simulink model "BPSK_FS_CFO_STO_finial"  (R2014b)
settings: Solver=VariableStepDiscrete  StartTime=0.0  StopTime=inf  RelTol=1e-3
values from neighbouring files (symbols this model uses):
  L = length(corr)    [barkerBits.m]
undefined symbols (not defined in the file or in its folder): alpha, del_f, dfilt, jsin, N, timing_offset, Ts
libraries: commnoisgen2 x4, commdigbbndpm3 x2, dspindex x2, dspobslib x2, dspsigops x2, commfilt2 x2, commchan3 x1, commrandsrc2 x1, simulink x1, commsink2 x1
settings Model: Creator=magarini_2  LastModifiedBy=magarini_2
settings OptimizationCC: UseDivisionForNetSlopeComputation=off  SimCompilerOptimization=off
settings DebuggingCC: FrameProcessingCompatibilityMsg=error
settings RTWCC: RTWCompilerOptimization=off

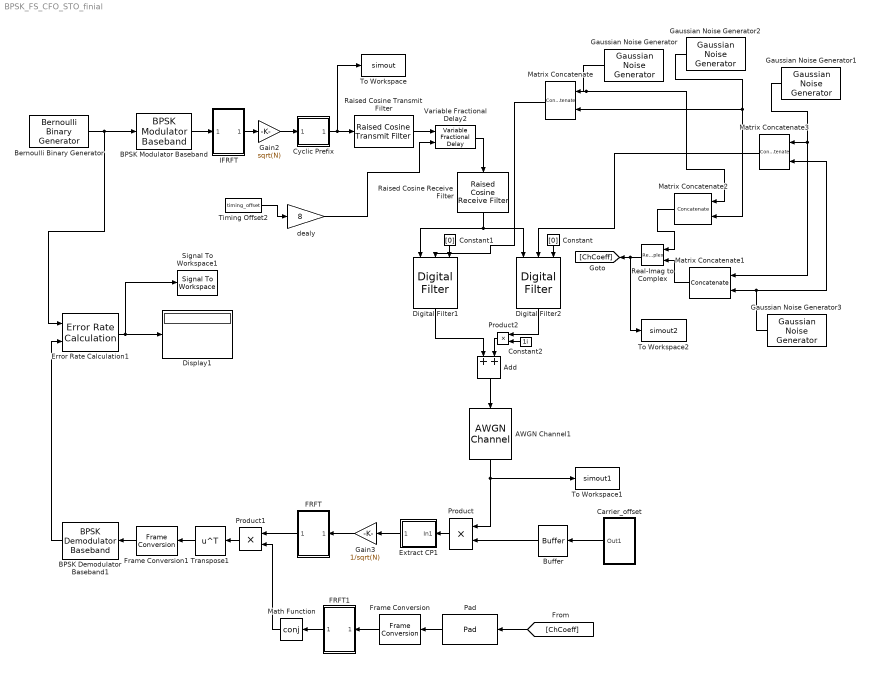
== system BPSK_FS_CFO_STO_finial ==
  AWGN Channel1 : commchan3/AWGN Channel  InputProcessing=Columns as channels (frame based)  seed=67  noiseMode="Signal to noise ratio  (SNR)"  EbNodB=50  EsNodB=10  SNRdB=SNR  bitsPerSym=1  Ps=1  Tsym=1  variance=1
  Add : Sum
  BPSK Demodulator Baseband1 : commdigbbndpm3/BPSK Demodulator Baseband  Ph=0  DecType=Hard decision  VarSource=Dialog  Variance=1  outDtype=Inherit via internal rule  derotateFactorWordLen=16
  BPSK Modulator Baseband : commdigbbndpm3/BPSK Modulator Baseband  Ph=0  outDtype=double  outWordLen=16  outUDDataType=sfix(16)  outFracLenMode=Best precision  outFracLen=15
  Bernoulli Binary Generator : commrandsrc2/Bernoulli Binary Generator  P=.5  seed=1361  Ts=Ts/N  frameBased=on  sampPerFrame=N  orient=off  outDataType=double
  Buffer : Buffer  N=N+L  TreatMby1Signals=One channel
  Carrier_offset : Subsystem
  Constant : Constant  Value=[0]  VectorParams1D=off  FramePeriod=1
      settings: SamplingMode=Frame based
  Constant1 : Constant  Value=[0]  VectorParams1D=off  FramePeriod=1
      settings: SamplingMode=Frame based
  Constant2 : Constant  Value=1i
  Cyclic Prefix : Subsystem
      mask Display: disp('CP')
  Digital Filter1 : dspobslib/Digital Filter  TypePopup=IIR (poles & zeros)  IIRFiltStruct=Direct form II transposed  AllPoleFiltStruct=Direct form  FIRFiltStruct=Direct form  CoeffSource=Input port(s)  NumCoeffs=randn  DenCoeffs=[1 1]  BiQuadCoeffs=[1 0.3 0.4 1 0.1 0.2]  LatticeCoeffs=[0.2 0.4]  denIgnore=on  FiltPerSampPopup=One filter per frame  IC=0  ICnum=0  ICden=0  roundingMode=Floor  overflowMode=off  ScaleValues=1  scaleValueFracLength=14  stageInFracLength=15  stageOutFracLength=15  FilterSource=Input port(s)  dfiltObjectName=dfilt.dffir([1 2 1])  InputProcessing=Columns as channels (frame based)
  Digital Filter2 : dspobslib/Digital Filter  TypePopup=IIR (poles & zeros)  IIRFiltStruct=Direct form II transposed  AllPoleFiltStruct=Direct form  FIRFiltStruct=Direct form  CoeffSource=Input port(s)  NumCoeffs=randn  DenCoeffs=[1 1]  BiQuadCoeffs=[1 0.3 0.4 1 0.1 0.2]  LatticeCoeffs=[0.2 0.4]  denIgnore=on  FiltPerSampPopup=One filter per frame  IC=0  ICnum=0  ICden=0  roundingMode=Floor  overflowMode=off  ScaleValues=1  scaleValueFracLength=14  stageInFracLength=15  stageOutFracLength=15  FilterSource=Input port(s)  dfiltObjectName=dfilt.dffir([1 2 1])  InputProcessing=Columns as channels (frame based)
  Display1 : Display
  Error Rate Calculation1 : commsink2/Error Rate Calculation  N=N  st_delay=N  cp_mode=Entire frame  subframe=[]  PMode=Port  WsName=ErrorVec  RsMode2=off  stop=on  numErr=maxNumErrs  maxBits=maxNumBits
  Extract CP1 : Subsystem
      mask Display: disp('CP^{-1}')
  FRFT : Subsystem
  FRFT1 : Subsystem
  Frame Conversion : FrameConversion  OutFrame=Sample-based
  Frame Conversion1 : FrameConversion
  Gain2 : Gain  Gain=sqrt(N)  OutDataTypeStr=double
  Gain3 : Gain  Gain=1/sqrt(N)
  Gaussian Noise Generator : commnoisgen2/Gaussian Noise Generator  m=0  d=1/4  s=1772  Ts=1  frameBased=on  sampPerFrame=1  orient=off  outDataType=double
  Gaussian Noise Generator1 : commnoisgen2/Gaussian Noise Generator  m=0  d=1/4  s=12313  Ts=1  frameBased=on  sampPerFrame=1  orient=off  outDataType=double
  Gaussian Noise Generator2 : commnoisgen2/Gaussian Noise Generator  m=0  d=1/4  s=14123  Ts=1  frameBased=on  sampPerFrame=1  orient=off  outDataType=double
  Gaussian Noise Generator3 : commnoisgen2/Gaussian Noise Generator  m=0  d=1/4  s=6632  Ts=1  frameBased=on  sampPerFrame=1  orient=off  outDataType=double
  IFRFT : Subsystem
  Math Function : Math  Operator=conj  SaturateOnIntegerOverflow=on
  Matrix Concatenate : Concatenate  Mode=Multidimensional array
  Matrix Concatenate1 : Concatenate  Mode=Multidimensional array  ConcatenateDimension=2
  Matrix Concatenate2 : Concatenate  Mode=Multidimensional array  ConcatenateDimension=2
  Matrix Concatenate3 : Concatenate  Mode=Multidimensional array
  Pad : dspsigops/Pad  padAlong=Rows  dimsToPad=1  valSrc=Specify via dialog  padVal=0  spec=Output size  padNumOutRowsSpecMethod=User-specified  numOutRows=8  padNumOutColsSpecMethod=User-specified  numOutCols=N  isVarDimsMode=off  padBeginning=0  padEnd=0  outSizeMode=User-specified  outSize=1  padSigAt=End  trunc_flag=None  roundingMode=Floor  overflowMode=off  truncOrWrapMode=Truncate  wrap_flag=None
  Product : Product
  Product1 : Product
  Product2 : Product
  Raised Cosine Receive Filter : commfilt2/Raised Cosine Receive Filter  filtType=Square root  N=10  filtSpan=N+L  currentFiltSpan=N+L  D=(N+L)/2  R=0.5  sampMode=Mute  saveAsFlag=0  rateMode=Downsampling  downFactor=10  downOffset=0  framing=Enforce single-rate processing  InputProcessing=Columns as channels (frame based)  checkGain=Normalized  filterGain=1  checkCoeff=on  variableName=rcRxFilt  launchFVT=on  roundingMode=Floor  overflowMode=off
  Raised Cosine Transmit Filter : commfilt2/Raised Cosine Transmit Filter  filtType=Square root  filtSpan=N+L  currentFiltSpan=N+L  D=(N+L)/2  R=0.5  sampMode=Mute  saveAsFlag=0  N=10  framing=Enforce single-rate processing  InputProcessing=Columns as channels (frame based)  checkGain=Normalized  filterGain=1  checkCoeff=on  variableName=rcTxFilt  launchFVT=on  roundingMode=Floor  overflowMode=off
  Real-Imag to Complex : RealImagToComplex
  Signal To Workspace1 : SignalToWorkspace  VariableName=SER1
      settings: CopyFcn=dspblkcopystw(gcbh);  MaxDataPoints=1
  Timing Offset2 : Constant  Value=timing_offset
  To Workspace : ToWorkspace  VariableName=simout  SaveFormat=Timeseries  SampleTime=-1
  To Workspace1 : ToWorkspace  VariableName=simout1  SaveFormat=Timeseries  SampleTime=-1
  To Workspace2 : ToWorkspace  VariableName=simout2  SaveFormat=Timeseries  SampleTime=-1
  Transpose1 : Math  Operator=transpose  SaturateOnIntegerOverflow=on
  Variable Fractional Delay2 : dspsigops/Variable Fractional Delay  mode=OBSOLETE  modeActive=Linear  dmax=10  InputProcessing=Columns as channels (frame based)  L=4  FarrowL=4  R=10  alpha=1  ic=0  fallbackFIR=Clip to the minimum value necessary for centered kernel  fallbackFarrow=Clip to the minimum value necessary for centered kernel  noDFT=off  roundingMode=Zero  overflowMode=off
  "dealy " : Gain  Gain=8  SaturateOnIntegerOverflow=on  OutDataTypeStr=Inherit: Same as input  ParamDataTypeStr=Inherit: Same as input
  wires:
  Frame Conversion1/1 -> BPSK Demodulator Baseband1/1
  Error Rate Calculation1/1 -> Signal To Workspace1/1, Display1/1
  BPSK Demodulator Baseband1/1 -> Error Rate Calculation1/2
  BPSK Modulator Baseband/1 -> IFRFT/1(In1)
  Buffer/1 -> Product/2
  Carrier_offset/1(Out1) -> Buffer/1
  IFRFT/1(Out1) -> Gain2/1
  Product/1 -> Extract CP1/1(In1)
  Gain2/1 -> Cyclic Prefix/1(In2)
  Gain3/1 -> FRFT/1(In1)
  Extract CP1/1(Out1) -> Gain3/1
  Cyclic Prefix/1(Out2) -> To Workspace/1, Raised Cosine Transmit Filter/1
  Transpose1/1 -> Frame Conversion1/1
  Gaussian Noise Generator1/1 -> Matrix Concatenate1/1, Matrix Concatenate3/1
  Gaussian Noise Generator/1 -> Matrix Concatenate2/1, Matrix Concatenate/1
  Matrix Concatenate/1 -> Digital Filter1/2
  Digital Filter1/1 -> Add/1
  Constant/1 -> Digital Filter2/3
  Constant1/1 -> Digital Filter1/3
  Real-Imag to Complex/1 -> To Workspace2/1, [ChCoeff]
  Digital Filter2/1 -> Product2/1
  Product2/1 -> Add/2
  Constant2/1 -> Product2/2
  [ChCoeff] -> Pad/1
  Pad/1 -> Frame Conversion/1
  FRFT1/1(Out1) -> Math Function/1
  Frame Conversion/1 -> FRFT1/1(In1)
  FRFT/1(Out1) -> Product1/1
  Product1/1 -> Transpose1/1
  Bernoulli Binary Generator/1 -> BPSK Modulator Baseband/1, Error Rate Calculation1/1
  Matrix Concatenate2/1 -> Real-Imag to Complex/1
  Matrix Concatenate3/1 -> Digital Filter2/2
  Matrix Concatenate1/1 -> Real-Imag to Complex/2
  Math Function/1 -> Product1/2
  Gaussian Noise Generator2/1 -> Matrix Concatenate2/2, Matrix Concatenate/2
  Gaussian Noise Generator3/1 -> Matrix Concatenate3/2, Matrix Concatenate1/2
  Raised Cosine Receive Filter/1 -> Digital Filter1/1, Digital Filter2/1
  Add/1 -> AWGN Channel1/1
  AWGN Channel1/1 -> Product/1, To Workspace1/1
  "dealy "/1 -> Variable Fractional Delay2/2
  Timing Offset2/1 -> "dealy "/1
  Raised Cosine Transmit Filter/1 -> Variable Fractional Delay2/1
  Variable Fractional Delay2/1 -> Raised Cosine Receive Filter/1

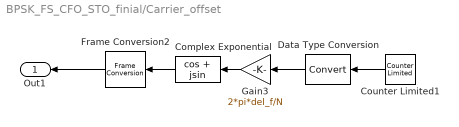
== system BPSK_FS_CFO_STO_finial/Carrier_offset ==
  Complex Exponential : Trigonometry  Operator=cos + jsin
  Counter Limited1 : simulink/Sources/Counter Limited  uplimit=N+L  tsamp=Ts/(N+L)
  Data Type Conversion : DataTypeConversion
  Frame Conversion2 : FrameConversion
  Gain3 : Gain  Gain=2*pi*del_f/N
  Out1 : Outport
  wires:
  Gain3/1 -> Complex Exponential/1
  Counter Limited1/1 -> Data Type Conversion/1
  Frame Conversion2/1 -> Out1/1
  Complex Exponential/1 -> Frame Conversion2/1
  Data Type Conversion/1 -> Gain3/1

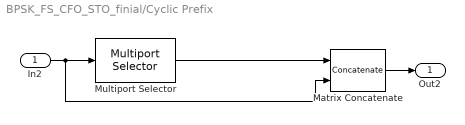
== system BPSK_FS_CFO_STO_finial/Cyclic Prefix ==
  In2 : Inport
  Matrix Concatenate : Concatenate  Mode=Multidimensional array
  Multiport Selector : dspindex/Multiport Selector  rowsOrCols=Rows  idxCellArray={ N-L+1:N }  idxErrMode=Clip Index
  Out2 : Outport
  wires:
  In2/1 -> Matrix Concatenate/2, Multiport Selector/1
  Multiport Selector/1 -> Matrix Concatenate/1
  Matrix Concatenate/1 -> Out2/1

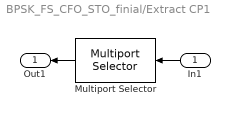
== system BPSK_FS_CFO_STO_finial/Extract CP1 ==
  In1 : Inport
  Multiport Selector : dspindex/Multiport Selector  rowsOrCols=Rows  idxCellArray={ (L+1):(N+L) }  idxErrMode=Clip Index
  Out1 : Outport
  wires:
  Multiport Selector/1 -> Out1/1
  In1/1 -> Multiport Selector/1

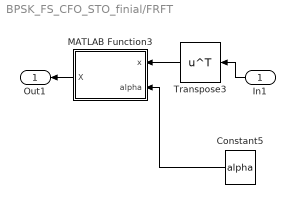
== system BPSK_FS_CFO_STO_finial/FRFT ==
  In1 : Inport
  Constant5 : Constant  Value=alpha  VectorParams1D=off
      settings: SamplingMode=Frame based
  MATLAB Function3 : MATLAB Function  TreatAsAtomicUnit=on
  Transpose3 : Math  Operator=transpose  SaturateOnIntegerOverflow=on
  Out1 : Outport
  wires:
  MATLAB Function3/1(X) -> Out1/1
  Transpose3/1 -> MATLAB Function3/1(x)
  Constant5/1 -> MATLAB Function3/2(alpha)
  In1/1 -> Transpose3/1

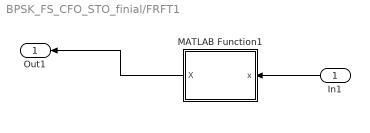
== system BPSK_FS_CFO_STO_finial/FRFT1 ==
  In1 : Inport
  MATLAB Function1 : MATLAB Function  TreatAsAtomicUnit=on
  Out1 : Outport
  wires:
  MATLAB Function1/1(X) -> Out1/1
  In1/1 -> MATLAB Function1/1(x)

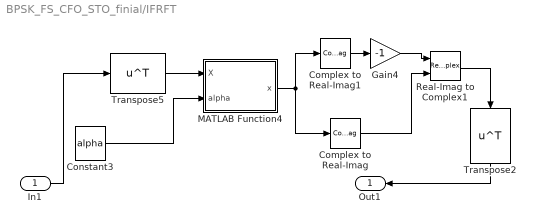
== system BPSK_FS_CFO_STO_finial/IFRFT ==
  In1 : Inport
  Complex to Real-Imag : ComplexToRealImag  Output=Real
  Complex to Real-Imag1 : ComplexToRealImag  Output=Imag
  Constant3 : Constant  Value=alpha  VectorParams1D=off
      settings: SamplingMode=Frame based
  Gain4 : Gain  Gain=-1
  MATLAB Function4 : MATLAB Function  TreatAsAtomicUnit=on
  Real-Imag to Complex1 : RealImagToComplex
  Transpose2 : Math  Operator=transpose  SaturateOnIntegerOverflow=on
  Transpose5 : Math  Operator=transpose  SaturateOnIntegerOverflow=on
  Out1 : Outport
  wires:
  MATLAB Function4/1(x) -> Complex to Real-Imag1/1, Complex to Real-Imag/1
  In1/1 -> Transpose5/1
  Gain4/1 -> Real-Imag to Complex1/1
  Transpose5/1 -> MATLAB Function4/1(X)
  Complex to Real-Imag/1 -> Real-Imag to Complex1/2
  Complex to Real-Imag1/1 -> Gain4/1
  Transpose2/1 -> Out1/1
  Constant3/1 -> MATLAB Function4/2(alpha)
  Real-Imag to Complex1/1 -> Transpose2/1

== matlab function BPSK_FS_CFO_STO_finial/FRFT1/MATLAB Function1 ==
  data: x input; X output
function X =atul_frft(x)
N=length(x);
% for alpha= 1.5:.001: 1.6
alpha =pi/2;
% alpha = 1.592;
a=alpha*2/pi;
A = sqrt((sin(alpha) - 1i*cos(alpha))/N);
delta_t=1;
delta_u =( 2*pi*abs(sin(alpha)) ) /(N);
n=0:1:N-1;
k=n;
kernel_frft = A*(exp(0.5*1i*cot(alpha)*(n.^2)'*(delta_t^2)) * exp(0.5*1i*cot(alpha)*(k.^2)*(delta_u^2)).* exp(-1i*2*pi*(n'*k)/N));
 X1 = x* kernel_frft;
 X=X1*sqrt(length(x));
end
% end

== matlab function BPSK_FS_CFO_STO_finial/FRFT/MATLAB Function3 ==
  data: x input; X output; alpha input
function X =atul_frft(x,alpha)
N=length(x);
a=alpha*2/pi;
A = sqrt((sin(alpha) - 1i*cos(alpha))/N);
delta_t=1;
delta_u =( 2*pi*abs(sin(alpha)) ) /(N);
n=0:1:N-1;
k=n;
kernel_frft = A*(exp(0.5*1i*cot(alpha)*(n.^2)'*(delta_t^2)) * exp(0.5*1i*cot(alpha)*(k.^2)*(delta_u^2)).* exp(-1i*2*pi*(n'*k)/N));
 X1 = x* kernel_frft;
 X=X1*sqrt(length(x));
end

== matlab function BPSK_FS_CFO_STO_finial/IFRFT/MATLAB Function4 ==
  data: X input; x output; alpha input
function x = atul_ifrft(X,alpha)
N=length(X);
a=alpha*2/pi;
A = sqrt((sin(alpha) - 1i*cos(alpha))/N);
delta_t=1;
delta_u = ( 2*pi*abs(sin(alpha)) ) /(N);
n=0:1:N-1;
k=n;
kernel_ifrft = -1i*A*(exp(0.5*1i*cot(alpha)*(n.^2)'*(delta_u^2)) * exp(0.5*1i*cot(alpha)*(k.^2)*(delta_t^2)).* exp(1i*2*pi*(n'*k)/N));
x = X * kernel_ifrft;
x=x/sqrt(length(X));
end
